simulink model "robot_joint_controlled_3_state"  (R2017b)
settings: Solver=ode8  StartTime=0.0  StopTime=2.0  FixedStep=0.00001  RelTol=1e-3
model workspace: external: MATLAB File D:\Projects\SERTS\Body\v7.0\Matlab\robot_DataFile.m (data not in the file)
values from neighbouring files (symbols this model uses):
  c_roll = 60    [best_so_far_variables.m]    (also in variables.m = 50)
  c_stance = [30,   0,    0 ... (first row only)    [best_so_far_variables.m]    (also in variables.m)
  c_swing = [50,   0,    0 ... (first row only)    [best_so_far_variables.m]    (also in variables.m = [100,   0,    0)
  c_yaw = 60    [best_so_far_variables.m]    (also in variables.m = 30)
  desired_body_height = 0.6    [best_so_far_variables.m]    (also in variables.m)
  desired_body_x_velocity = 0    [best_so_far_variables.m]    (also in variables.m)
  desired_body_y_velocity = 1    [best_so_far_variables.m]    (also in variables.m)
  desired_yaw = 0    [best_so_far_variables.m]    (also in variables.m)
  k_roll = 300    [best_so_far_variables.m]    (also in variables.m = 700)
  k_stance = [    0,    0,       0 ... (first row only)    [best_so_far_variables.m]    (also in variables.m)
  k_swing = [ 1000,     0,       0 ... (first row only)    [best_so_far_variables.m]    (also in variables.m = [02000,     0,       0)
  k_x = 0.03    [best_so_far_variables.m]    (also in variables.m)
  k_y = 0.03    [best_so_far_variables.m]    (also in variables.m)
  k_yaw = 300    [best_so_far_variables.m]    (also in variables.m)
  Left = 1    [best_so_far_variables.m]    (also in variables.m)
  LF_RH = -1    [best_so_far_variables.m]    (also in variables.m)
  lift_height = 0.05    [best_so_far_variables.m]    (also in variables.m)
  RF_LH = 1    [best_so_far_variables.m]    (also in variables.m)
  Right = -1    [best_so_far_variables.m]    (also in variables.m)
  stance_time = 0.2    [best_so_far_variables.m]    (also in variables.m)
  weight = 19    [best_so_far_variables.m]    (also in variables.m)
  width = 0.375    [best_so_far_variables.m]    (also in variables.m)
undefined symbols (not defined in the file or in its folder): smiData, X, Y, Z
libraries: sm_lib x1540, nesl_utility x44, Contact_Forces_Lib x4, simulink x4
(part 32 of 32)

== matlab function robot_joint_controlled_3_state/Leg_model_left_2/controller /MATLAB Function ==
  data: select input; pair_selector input; side_selector input; width input; weight input; k_swing input; c_swing input; k_stance input; c_stance input; k_roll input; c_roll input; k_yaw input; c_yaw input; yaw input; desired_yaw input; yaw_rate input; roll input; roll_rate input; x_sw input; y_sw input; z_sw input; desired_body_height input; body_x_velocity input; body_y_velocity input; body_z_velocity input; desired_body_x_velocity input; desired_body_y_velocity input; T1 output; T2 output; T3 output; theta_1 input; theta_2 input; theta_3 input; theta_1_rate input; theta_2_rate input; theta_3_rate input
function [T1, T2, T3] = VMC_Controller(select, pair_selector, side_selector, width, weight, k_swing, c_swing, k_stance, c_stance, k_roll, c_roll, k_yaw, c_yaw, yaw, desired_yaw, yaw_rate, roll, roll_rate, x_sw, y_sw, z_sw, desired_body_height, body_x_velocity, body_y_velocity, body_z_velocity, desired_body_x_velocity, desired_body_y_velocity, theta_1, theta_2, theta_3, theta_1_rate, theta_2_rate, theta_3_rate)


jacobian = [    -0.310*cos(theta_1)*cos(theta_2-theta_3)-0.255*cos(theta_1)*cos(theta_2)-0.14*cos(theta_1),     0.310*sin(theta_1)*sin(theta_2-theta_3)+0.255*sin(theta_1)*sin(theta_2),    -0.310*sin(theta_1)*sin(theta_2-theta_3);
                 0,                                                                                            -0.310*cos(theta_2-theta_3)-0.255*cos(theta_2),                               0.310*cos(theta_2-theta_3);
                 0.310*sin(theta_1)*cos(theta_2-theta_3)+0.255*sin(theta_1)*cos(theta_2)+0.14*sin(theta_1),     0.310*cos(theta_1)*sin(theta_2-theta_3)+0.255*cos(theta_1)*sin(theta_2),    -0.310*cos(theta_1)*sin(theta_2-theta_3)    ];
      
             
x = -0.310*sin(theta_1)*cos(theta_2-theta_3)-0.255*sin(theta_1)*cos(theta_2)-0.14*sin(theta_1);
y = -0.310*sin(theta_2-theta_3)-0.255*sin(theta_2);
z = -0.310*cos(theta_1)*cos(theta_2-theta_3)-0.255*cos(theta_1)*cos(theta_2)-0.14*cos(theta_1);
   
joint_velocity = [  theta_1_rate;
                    theta_2_rate;
                    theta_3_rate ];

foot_velocity = jacobian*joint_velocity;

x_rate = foot_velocity(1);
y_rate = foot_velocity(2);
z_rate = foot_velocity(3);


if select>0
    
    delta_T = -0.5*((k_roll*roll) + (c_roll*roll_rate));
    
    delta_f = ((k_yaw*(desired_yaw - yaw)) - (c_yaw*yaw_rate)) / width;
    
    position_vector = [ (-1*x);
                        (-1*y);
                        ((weight*9.81/k_stance(3,3)) + desired_body_height + z) ];
    
    velocity_vector = [ (desired_body_x_velocity - body_x_velocity);
                        (desired_body_y_velocity - body_y_velocity);
                        ( -1*body_z_velocity) ];
                    
    force_vector = [    0;
                        (pair_selector*delta_f);
                        0 ];
                    
    torque_vector = [   (side_selector*delta_T);
                        0;
                        0 ];
                    
    force = (k_stance*position_vector) + (c_stance*velocity_vector) + force_vector;
    
    torque = -1*transpose(jacobian)*force - torque_vector;
                    
else
    
    position_vector = [ (x_sw - x);
                        (y_sw - y);
                        (z_sw - z) ];
    
    velocity_vector = [ (-1*x_rate);
                        (-1*y_rate);
                        (-1*z_rate)];
                        
    force = ((k_swing*position_vector) + (c_swing*velocity_vector));
    
    torque = transpose(jacobian)*force;
    
end

T1 = torque(1);
T2 = torque(2);
T3 = torque(3);

== matlab function robot_joint_controlled_3_state/Leg_model_left_2/controller /MATLAB Function1 ==
  data: k_x input; x_sw output; k_y input; desired_body_x_velocity input; desired_body_y_velocity input; body_x_velocity input; body_y_velocity input; lift_height input; time input; stance_time input; x_lo input; y_lo input; z_lo input; y_sw output; z_sw output
function [x_sw, y_sw, z_sw] = Trajectory_Generator(k_x, k_y, desired_body_x_velocity, desired_body_y_velocity, body_x_velocity, body_y_velocity, lift_height, time, stance_time, x_lo, y_lo, z_lo)

yf = ((0.5*body_y_velocity*stance_time) - (k_y*(desired_body_y_velocity - body_y_velocity)));
xf = ((0.5*body_x_velocity*stance_time) - (k_x*(desired_body_x_velocity - body_x_velocity)));

phi = (2*3.14*time)/stance_time;

x_sw = (x_lo + ((xf - x_lo)*(phi - sin(phi))/(2*3.14)));
y_sw = (y_lo + ((yf - y_lo)*(phi - sin(phi))/(2*3.14)));
z_sw = (z_lo + (lift_height*(1 - cos(phi))/2));

== stateflow chart robot_joint_controlled_3_state/Leg_model_right_2/controller /Chart ==
  state Set_State_Swing
    entry: x = -0.310*sin(theta_1)*cos(theta_2-theta_3)-0.255*sin(theta_1)*cos(theta_2)-0.14*sin(theta_1);
    y = -0.310*sin(theta_2-theta_3)-0.255*sin(theta_2);
    z = -0.310*cos(theta_1)*cos(theta_2-theta_3)-0.255*cos(theta_1)*cos(theta_2)-0.14*cos(theta_1);
  state Fixed_State_State
    entry: x = x
    y = y
    z = z
  (default) -> Set_State_Swing
  Set_State_Swing -> Fixed_State_State : [select == 1 ]
  Fixed_State_State -> Set_State_Swing : [select == 0]
  data: theta_1 input; theta_2 input; theta_3 input; select input; x output; y output; z output

== matlab function robot_joint_controlled_3_state/Leg_model_right_2/controller /MATLAB Function ==
  data: select input; pair_selector input; side_selector input; width input; weight input; k_swing input; c_swing input; k_stance input; c_stance input; k_roll input; c_roll input; k_yaw input; c_yaw input; yaw input; desired_yaw input; yaw_rate input; roll input; roll_rate input; x_sw input; y_sw input; z_sw input; desired_body_height input; body_x_velocity input; body_y_velocity input; body_z_velocity input; desired_body_x_velocity input; desired_body_y_velocity input; T1 output; T2 output; T3 output; theta_1 input; theta_2 input; theta_3 input; theta_1_rate input; theta_2_rate input; theta_3_rate input
function [T1, T2, T3] = VMC_Controller(select, pair_selector, side_selector, width, weight, k_swing, c_swing, k_stance, c_stance, k_roll, c_roll, k_yaw, c_yaw, yaw, desired_yaw, yaw_rate, roll, roll_rate, x_sw, y_sw, z_sw, desired_body_height, body_x_velocity, body_y_velocity, body_z_velocity, desired_body_x_velocity, desired_body_y_velocity, theta_1, theta_2, theta_3, theta_1_rate, theta_2_rate, theta_3_rate)


jacobian = [    -0.310*cos(theta_1)*cos(theta_2-theta_3)-0.255*cos(theta_1)*cos(theta_2)-0.14*cos(theta_1),     0.310*sin(theta_1)*sin(theta_2-theta_3)+0.255*sin(theta_1)*sin(theta_2),    -0.310*sin(theta_1)*sin(theta_2-theta_3);
                 0,                                                                                            -0.310*cos(theta_2-theta_3)-0.255*cos(theta_2),                               0.310*cos(theta_2-theta_3);
                 0.310*sin(theta_1)*cos(theta_2-theta_3)+0.255*sin(theta_1)*cos(theta_2)+0.14*sin(theta_1),     0.310*cos(theta_1)*sin(theta_2-theta_3)+0.255*cos(theta_1)*sin(theta_2),    -0.310*cos(theta_1)*sin(theta_2-theta_3)    ];
      
             
x = -0.310*sin(theta_1)*cos(theta_2-theta_3)-0.255*sin(theta_1)*cos(theta_2)-0.14*sin(theta_1);
y = -0.310*sin(theta_2-theta_3)-0.255*sin(theta_2);
z = -0.310*cos(theta_1)*cos(theta_2-theta_3)-0.255*cos(theta_1)*cos(theta_2)-0.14*cos(theta_1);
   
joint_velocity = [  theta_1_rate;
                    theta_2_rate;
                    theta_3_rate ];

foot_velocity = jacobian*joint_velocity;

x_rate = foot_velocity(1);
y_rate = foot_velocity(2);
z_rate = foot_velocity(3);


if select>0
    
    delta_T = -0.5*((k_roll*roll) + (c_roll*roll_rate));
    
    delta_f = ((k_yaw*(desired_yaw - yaw)) - (c_yaw*yaw_rate)) / width;
    
    position_vector = [ (-1*x);
                        (-1*y);
                        ((weight*9.81/k_stance(3,3)) + desired_body_height + z) ];
    
    velocity_vector = [ (desired_body_x_velocity - body_x_velocity);
                        (desired_body_y_velocity - body_y_velocity);
                        ( -1*body_z_velocity) ];
                    
    force_vector = [    0;
                        (pair_selector*delta_f);
                        0 ];
                    
    torque_vector = [   (side_selector*delta_T);
                        0;
                        0 ];
                    
    force = (k_stance*position_vector) + (c_stance*velocity_vector) + force_vector;
    
    torque = -1*transpose(jacobian)*force - torque_vector;
                    
else
    
    position_vector = [ (x_sw - x);
                        (y_sw - y);
                        (z_sw - z) ];
    
    velocity_vector = [ (-1*x_rate);
                        (-1*y_rate);
                        (-1*z_rate)];
                        
    force = ((k_swing*position_vector) + (c_swing*velocity_vector));
    
    torque = transpose(jacobian)*force;
    
end

T1 = torque(1);
T2 = torque(2);
T3 = torque(3);

== matlab function robot_joint_controlled_3_state/Leg_model_right_2/controller /MATLAB Function1 ==
  data: k_x input; x_sw output; k_y input; desired_body_x_velocity input; desired_body_y_velocity input; body_x_velocity input; body_y_velocity input; lift_height input; time input; stance_time input; x_lo input; y_lo input; z_lo input; y_sw output; z_sw output
function [x_sw, y_sw, z_sw] = Trajectory_Generator(k_x, k_y, desired_body_x_velocity, desired_body_y_velocity, body_x_velocity, body_y_velocity, lift_height, time, stance_time, x_lo, y_lo, z_lo)

yf = ((0.5*body_y_velocity*stance_time) - (k_y*(desired_body_y_velocity - body_y_velocity)));
xf = ((0.5*body_x_velocity*stance_time) - (k_x*(desired_body_x_velocity - body_x_velocity)));

phi = (2*3.14*time)/stance_time;

x_sw = (x_lo + ((xf - x_lo)*(phi - sin(phi))/(2*3.14)));
y_sw = (y_lo + ((yf - y_lo)*(phi - sin(phi))/(2*3.14)));
z_sw = (z_lo + (lift_height*(1 - cos(phi))/2));

== stateflow chart robot_joint_controlled_3_state/Chart ==
  state Intermediate1
    entry: LF = 2
    RF = 1
    RH = 0
    LH = 1
  state Intermediate
    entry: LF = 0
    RF = 1
    RH = 2
    LH = 1
  state LF_RH_swing
    entry: LF = 0
    RF = 1
    RH = 0
    LH = 1
  state RF_LH_swing
    entry: LF = 1
    RF = 0
    RH = 1
    LH = 0
  state Intermediate3
    entry: LF = 1
    RF = 0
    RH = 1
    LH = 2
  state Intermediate2
    entry: LF = 1
    RF = 2
    RH = 1
    LH = 0
  LF_RH_swing -> Intermediate1 [order 1] : [LFS*pulse]
  Intermediate1 -> RF_LH_swing : [RHS*pulse]
  Intermediate -> RF_LH_swing : [LFS*pulse]
  LF_RH_swing -> Intermediate [order 2] : [RHS*pulse]
  (default) -> LF_RH_swing
  Intermediate3 -> LF_RH_swing : [RFS*pulse]
  RF_LH_swing -> Intermediate3 [order 2] : [LHS*pulse]
  Intermediate2 -> LF_RH_swing : [LHS*pulse]
  RF_LH_swing -> Intermediate2 [order 1] : [RFS*pulse]
  data: LF output; LH output; RF output; RH output; LFS input; LHS input; RHS input; RFS input; pulse input

== matlab function robot_joint_controlled_3_state/Leg_model_right_2/Subsystem/MATLAB Function ==
  data: normal_force input; touch output
function touch = TouchIdentifier(normal_force)

if normal_force>0
    touch = 1;
else
    touch = 0;
end

== matlab function robot_joint_controlled_3_state/Leg_model_left_1/Subsystem/MATLAB Function ==
  data: normal_force input; touch output
function touch = TouchIdentifier(normal_force)

if normal_force>0
    touch = 1;
else
    touch = 0;
end

== matlab function robot_joint_controlled_3_state/Leg_model_left_2/Subsystem/MATLAB Function ==
  data: normal_force input; touch output
function touch = TouchIdentifier(normal_force)

if normal_force>0
    touch = 1;
else
    touch = 0;
end

== matlab function robot_joint_controlled_3_state/Leg_model_right_1/Subsystem/MATLAB Function ==
  data: normal_force input; touch output
function touch = TouchIdentifier(normal_force)

if normal_force>0
    touch = 1;
else
    touch = 0;
end
